simulink model "ulohaStyri_simulink"  (R2022b)
settings: Solver=VariableStepAuto  StartTime=0.0  StopTime=60  RelTol=1e-3
model workspace (MAT data in the model file):
  a0 = -5
  a1 = -4
  a2 = 1
settings Model: Creator=marak  LastModifiedBy=marak

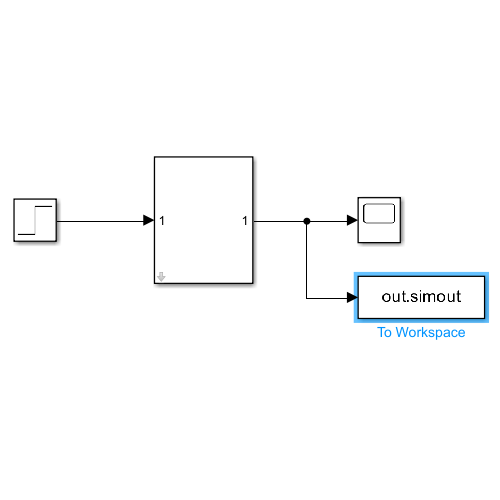
[thumbnail: Simulink's stored preview of the top-level diagram]
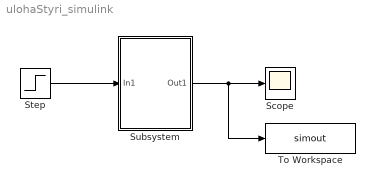
== system ulohaStyri_simulink ==
  Scope : Scope
  Step : Step  SampleTime=0
  Subsystem : Subsystem  mask{m=1, k=1, b=0.2}
  To Workspace : ToWorkspace  VariableName=simout  SaveFormat=Timeseries  SampleTime=-1
  wires:
  Step/1 -> Subsystem/1(In1)
  Subsystem/1(Out1) -> To Workspace/1, Scope/1

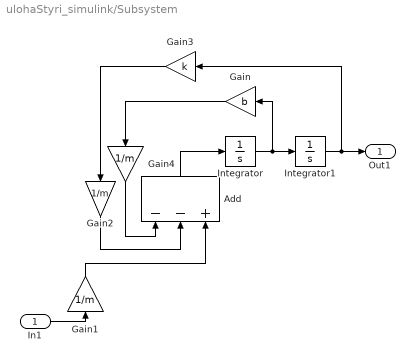
== system ulohaStyri_simulink/Subsystem ==
  In1 : Inport
  Add : Sum  Inputs=--+
  Gain : Gain  Gain=b
  Gain1 : Gain  Gain=1/m
  Gain2 : Gain  Gain=1/m
  Gain3 : Gain  Gain=k
  Gain4 : Gain  Gain=1/m
  Integrator : Integrator
  Integrator1 : Integrator
  Out1 : Outport
  wires:
  In1/1 -> Gain1/1
  Gain1/1 -> Add/3
  Integrator/1 -> Integrator1/1, Gain/1
  Add/1 -> Integrator/1
  Gain2/1 -> Add/2
  Gain3/1 -> Gain2/1
  Gain/1 -> Gain4/1
  Gain4/1 -> Add/1
  Integrator1/1 -> Out1/1, Gain3/1
